simulink model "uz_typeconv_multi"  (R2021a)
settings: Solver=FixedStepDiscrete  StartTime=0.0  StopTime=0.001  RelTol=1e-3
values from neighbouring files (symbols this model uses):
  t_ADC = 1/f_ADC    (= 1e-05)    [uz_6ph_pu_vsd_voltages_init.m]    (also in uz_mpc_6ph_init.m; uz_mpc_6ph_state_machine_init.m; uz_typeconv_init.m)
libraries: simulink x1
settings Model: DataTypeOverride=Off  Creator=micha  LastModifiedBy=micha
settings SolverCC: AlgebraicLoopSolver=TrustRegion
settings DataIOCC: LimitDataPoints=on  SaveOutput=off  SaveTime=off
settings OptimizationCC: BlockReduction=off  ConditionallyExecuteInputs=off  DefaultParameterBehavior=Inlined  LifeSpan=inf
settings DebuggingCC: AlgebraicLoopMsg=error  SingleTaskRateTransMsg=error  AllowSymbolicDim=off  StrictBusMsg=ErrorOnBusTreatedAsVector  SFUnexpectedBacktrackingDiag=warning  SFNoUnconditionalDefaultTransitionDiag=warning  SFExecutionAtInitializationDiag=none  SFMachineParentedDataDiag=warning  ArithmeticOperatorsInVariantConditions=warning
settings HardwareCC: ProdBitPerPointer=32  ProdBitPerSizeT=32  ProdBitPerPtrDiffT=32  ProdLargestAtomicFloat=None  ProdIntDivRoundTo=Undefined  ProdEndianess=Unspecified  ProdWordSize=32  ProdHWDeviceType=ASIC/FPGA->ASIC/FPGA  ProdEqTarget=off
settings SFSimCC: SimUseLocalCustomCode=off  CustomCodeUndefinedFunction=UseInterfaceOnly
settings RTWCC: RTWUseLocalCustomCode=off
settings CodeAppCC: StateflowObjectComments=on
settings GRTTargetCC: TargetLangStandard=C89/C90 (ANSI)
settings ConfigComp: CovScope=ReferencedModels  CovMetricSettings=dw  CovSaveCumulativeToWorkspaceVar=on  CovSaveSingleToWorkspaceVar=on  CovExternalEMLEnable=off  CovSFcnEnable=off

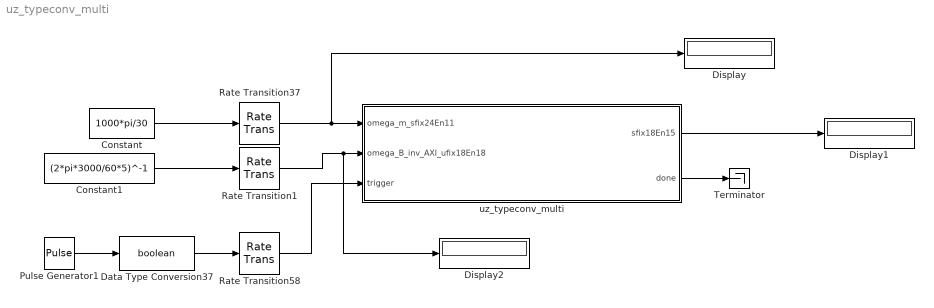
== system uz_typeconv_multi ==
  Constant : Constant  Value=1000*pi/30  OutDataTypeStr=fixdt(1,24,11)  SampleTime=-1
  Constant1 : Constant  Value=(2*pi*3000/60*5)^-1  OutDataTypeStr=fixdt(0,18,18)  SampleTime=-1
  Data Type Conversion37 : DataTypeConversion  OutDataTypeStr=boolean
  Display : Display
  Display1 : Display
  Display2 : Display
  Pulse Generator1 : DiscretePulseGenerator  PulseType=Time based  Period=t_ADC  PulseWidth=5
  Rate Transition1 : RateTransition  OutPortSampleTime=t_clock
  Rate Transition37 : RateTransition  OutPortSampleTime=t_clock
  Rate Transition58 : RateTransition  OutPortSampleTime=t_clock
  Terminator : Terminator
  uz_typeconv_multi : Subsystem  TreatAsAtomicUnit=on
  wires:
  Constant/1 -> Rate Transition37/1
  uz_typeconv_multi/1(sfix18En15) -> Display1/1
  Data Type Conversion37/1 -> Rate Transition58/1
  Pulse Generator1/1 -> Data Type Conversion37/1
  Rate Transition58/1 -> uz_typeconv_multi/3(trigger)
  Rate Transition37/1 -> Display/1, uz_typeconv_multi/1(omega_m_sfix24En11)
  uz_typeconv_multi/2(done) -> Terminator/1
  Constant1/1 -> Rate Transition1/1
  Rate Transition1/1 -> Display2/1, uz_typeconv_multi/2(omega_B_inv_AXI_ufix18En18)

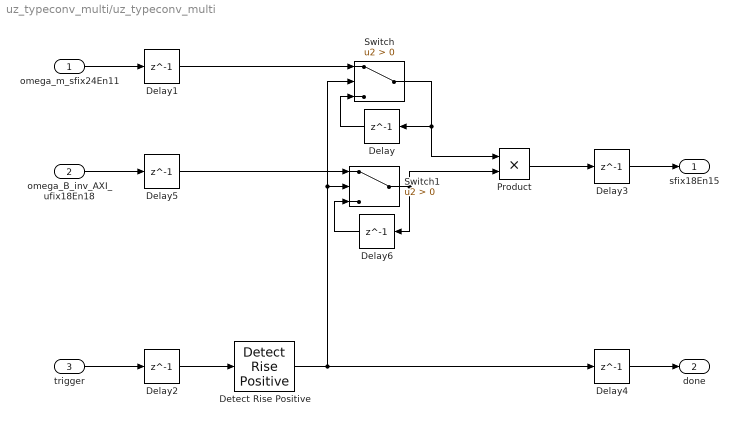
== system uz_typeconv_multi/uz_typeconv_multi ==
  omega_m_sfix24En11 : Inport
  omega_B_inv_AXI_ufix18En18 : Inport  Port=2
  trigger : Inport  Port=3
  Delay{,1..6} (7 alike) : Delay  DelayLength=1
  Detect Rise Positive : simulink/Logic and Bit Operations/Detect Rise Positive  vinit=0  OutDataTypeStr=boolean
  Product : Product  OutDataTypeStr=fixdt(1,18,15)
  Switch : Switch  Criteria=u2 > Threshold
  Switch1 : Switch  Criteria=u2 > Threshold
  sfix18En15 : Outport  VectorParamsAs1DForOutWhenUnconnected=off
  done : Outport  Port=2  VectorParamsAs1DForOutWhenUnconnected=off
  wires:
  Product/1 -> Delay3/1
  trigger/1 -> Delay2/1
  Detect Rise Positive/1 -> Switch1/2, Switch/2, Delay4/1
  Switch/1 -> Product/1, Delay/1
  Delay/1 -> Switch/3
  omega_m_sfix24En11/1 -> Delay1/1
  Delay1/1 -> Switch/1
  Delay2/1 -> Detect Rise Positive/1
  Delay3/1 -> sfix18En15/1
  Delay4/1 -> done/1
  Delay5/1 -> Switch1/1
  omega_B_inv_AXI_ufix18En18/1 -> Delay5/1
  Switch1/1 -> Product/2, Delay6/1
  Delay6/1 -> Switch1/3
